simulink library "xProdMatrix_ul"  (R2022a)
settings: Solver=VariableStepAuto  StartTime=0.0  StopTime=10.0  RelTol=1e-3
libraries: sharedutil x1
settings Model: Creator=jldanie5  LastModifiedBy=lhill8
settings SolverCC: AlgebraicLoopSolver=TrustRegion
settings DebuggingCC: UnconnectedInputMsg=warning  UnconnectedOutputMsg=warning  UnconnectedLineMsg=warning  SFMachineParentedDataDiag=warning  ArithmeticOperatorsInVariantConditions=warning
settings SFSimCC: CustomCodeUndefinedFunction=UseInterfaceOnly

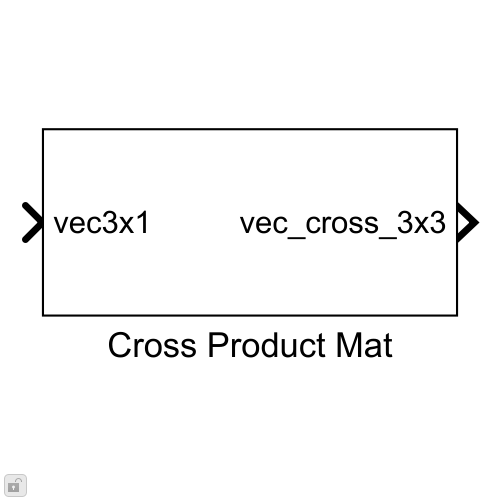
[thumbnail: Simulink's stored preview of the top-level diagram]
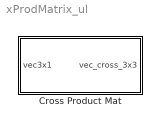
== system xProdMatrix_ul ==
  Cross Product Mat : Subsystem

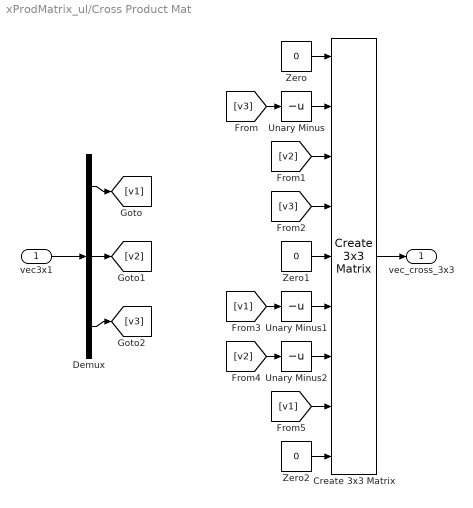
== system xProdMatrix_ul/Cross Product Mat ==
  vec3x1 : Inport
  Create 3x3 Matrix : sharedutil/Create 3x3 Matrix  aMode=aMode
      settings: SourceProductBaseCode=AE,PW,DR,MT,VE
  Demux : Demux  Outputs=3
  Unary Minus : UnaryMinus
  Unary Minus1 : UnaryMinus
  Unary Minus2 : UnaryMinus
  Zero : Constant  Value=0  OutDataTypeStr=Inherit: Inherit via back propagation
  Zero1 : Constant  Value=0  OutDataTypeStr=Inherit: Inherit via back propagation
  Zero2 : Constant  Value=0  OutDataTypeStr=Inherit: Inherit via back propagation
  vec_cross_3x3 : Outport  VectorParamsAs1DForOutWhenUnconnected=off
  wires:
  [v1] -> Create 3x3 Matrix/8
  [v2] -> Unary Minus2/1
  [v1] -> Unary Minus1/1
  [v3] -> Create 3x3 Matrix/4
  [v2] -> Create 3x3 Matrix/3
  [v3] -> Unary Minus/1
  Zero2/1 -> Create 3x3 Matrix/9
  Zero1/1 -> Create 3x3 Matrix/5
  Zero/1 -> Create 3x3 Matrix/1
  Unary Minus2/1 -> Create 3x3 Matrix/7
  Unary Minus1/1 -> Create 3x3 Matrix/6
  Unary Minus/1 -> Create 3x3 Matrix/2
  Demux/3 -> [v3]
  Demux/2 -> [v2]
  Demux/1 -> [v1]
  Create 3x3 Matrix/1 -> vec_cross_3x3/1
  vec3x1/1 -> Demux/1
